simulink library "INT_HLSDem_CalcState"  (R2016b)
settings: Solver=VariableStepAuto  StartTime=0.0  StopTime=10.0  RelTol=1e-3
settings Model: Creator=xuxingpei  LastModifiedBy=xuxingpei

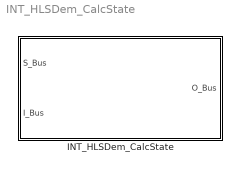
== system INT_HLSDem_CalcState ==
  INT_HLSDem_CalcState : Subsystem

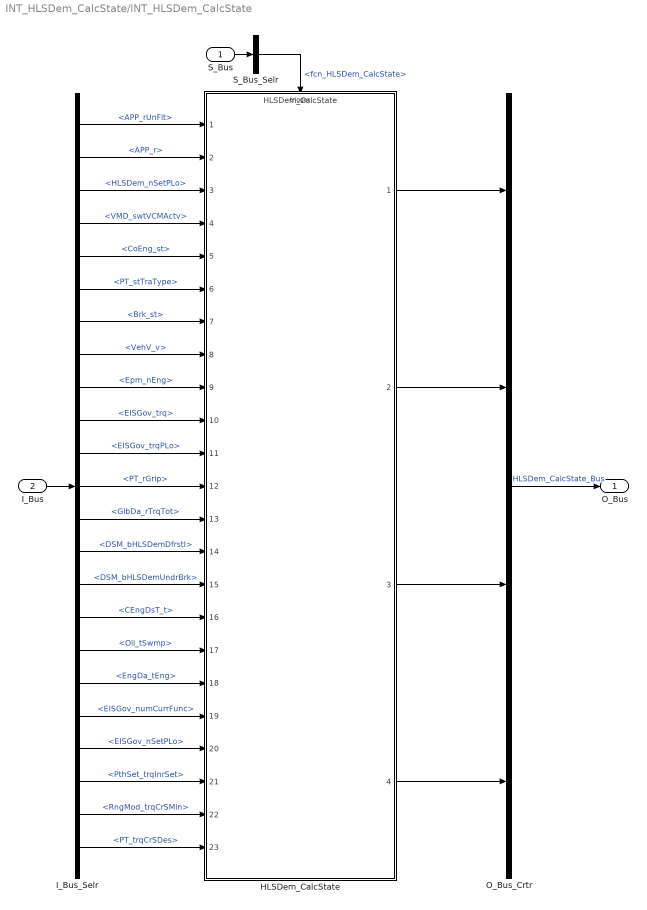
== system INT_HLSDem_CalcState/INT_HLSDem_CalcState ==
  S_Bus : Inport
  I_Bus : Inport  Port=2
  HLSDem_CalcState : ModelReference  ModelNameDialog=HLSDem_CalcState  SimulationMode=Normal  ModelReferenceVersion=1.139  TriggerPortName=function  TriggerPortTriggerType=function-call  TriggerPortStatesWhenEnabling=held
  I_Bus_Selr : BusSelector  OutputSignals=APP_rUnFlt,APP_r,HLSDem_nSetPLo,VMD_swtVCMActv,CoEng_st,PT_stTraType,Brk_st,VehV_v,Epm_nEng,EISGov_trq,EISGov_trqPLo,PT_rGrip,GlbDa_rTrqTot,DSM_bHLSDemDfrstI,DSM_bHLSDemUndrBrk,CEngDsT_t,Oil_tSwmp,EngDa_tEng,EISGov_numCurrFunc,EISGov_nSetPLo,PthSet_trqInrSet,RngMod_trqCrSMin,PT_trqCrSDes
  O_Bus_Crtr : BusCreator  Inputs=4
  S_Bus_Selr : BusSelector  OutputSignals=fcn_HLSDem_CalcState
  O_Bus : Outport
  wires:
  S_Bus_Selr/1 -> HLSDem_CalcState/Trigger  "<fcn_HLSDem_CalcState>"
  S_Bus/1 -> S_Bus_Selr/1
  I_Bus/1 -> I_Bus_Selr/1
  I_Bus_Selr/1 -> HLSDem_CalcState/1  "<APP_rUnFlt>"
  I_Bus_Selr/2 -> HLSDem_CalcState/2  "<APP_r>"
  I_Bus_Selr/3 -> HLSDem_CalcState/3  "<HLSDem_nSetPLo>"
  I_Bus_Selr/4 -> HLSDem_CalcState/4  "<VMD_swtVCMActv>"
  I_Bus_Selr/5 -> HLSDem_CalcState/5  "<CoEng_st>"
  I_Bus_Selr/6 -> HLSDem_CalcState/6  "<PT_stTraType>"
  I_Bus_Selr/7 -> HLSDem_CalcState/7  "<Brk_st>"
  I_Bus_Selr/8 -> HLSDem_CalcState/8  "<VehV_v>"
  I_Bus_Selr/9 -> HLSDem_CalcState/9  "<Epm_nEng>"
  I_Bus_Selr/10 -> HLSDem_CalcState/10  "<EISGov_trq>"
  I_Bus_Selr/11 -> HLSDem_CalcState/11  "<EISGov_trqPLo>"
  I_Bus_Selr/12 -> HLSDem_CalcState/12  "<PT_rGrip>"
  I_Bus_Selr/13 -> HLSDem_CalcState/13  "<GlbDa_rTrqTot>"
  I_Bus_Selr/14 -> HLSDem_CalcState/14  "<DSM_bHLSDemDfrstI>"
  I_Bus_Selr/15 -> HLSDem_CalcState/15  "<DSM_bHLSDemUndrBrk>"
  I_Bus_Selr/16 -> HLSDem_CalcState/16  "<CEngDsT_t>"
  I_Bus_Selr/17 -> HLSDem_CalcState/17  "<Oil_tSwmp>"
  I_Bus_Selr/18 -> HLSDem_CalcState/18  "<EngDa_tEng>"
  I_Bus_Selr/19 -> HLSDem_CalcState/19  "<EISGov_numCurrFunc>"
  I_Bus_Selr/20 -> HLSDem_CalcState/20  "<EISGov_nSetPLo>"
  I_Bus_Selr/21 -> HLSDem_CalcState/21  "<PthSet_trqInrSet>"
  I_Bus_Selr/22 -> HLSDem_CalcState/22  "<RngMod_trqCrSMin>"
  I_Bus_Selr/23 -> HLSDem_CalcState/23  "<PT_trqCrSDes>"
  O_Bus_Crtr/1 -> O_Bus/1  "HLSDem_CalcState_Bus"
  HLSDem_CalcState/1 -> O_Bus_Crtr/1
  HLSDem_CalcState/2 -> O_Bus_Crtr/2
  HLSDem_CalcState/3 -> O_Bus_Crtr/3
  HLSDem_CalcState/4 -> O_Bus_Crtr/4
